simulink model "oppg2b"  (R2024a)
settings: Solver=VariableStepAuto  StartTime=0.0  StopTime=10.0  RelTol=1e-3
settings Model: Creator=Lars André  LastModifiedBy=Lars André

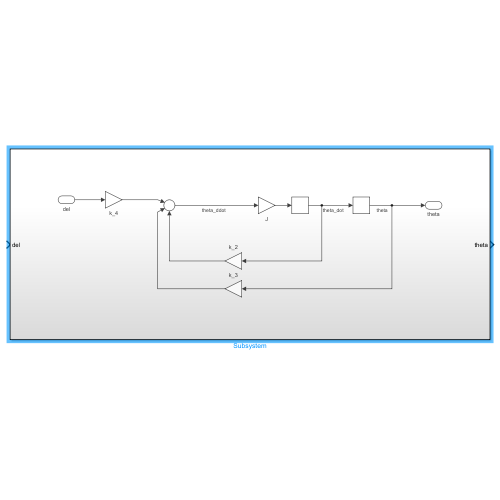
[thumbnail: Simulink's stored preview of the top-level diagram]
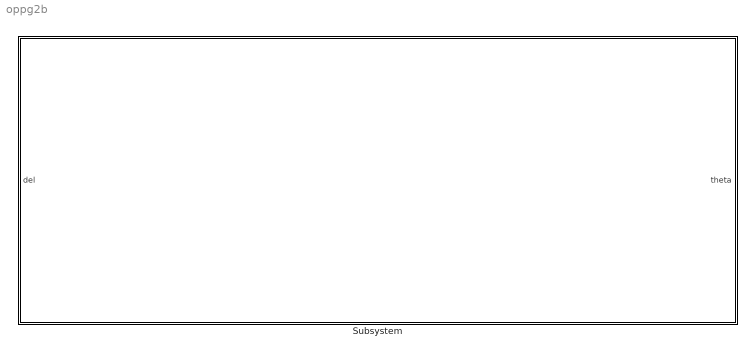
== system oppg2b ==
  Subsystem : Subsystem

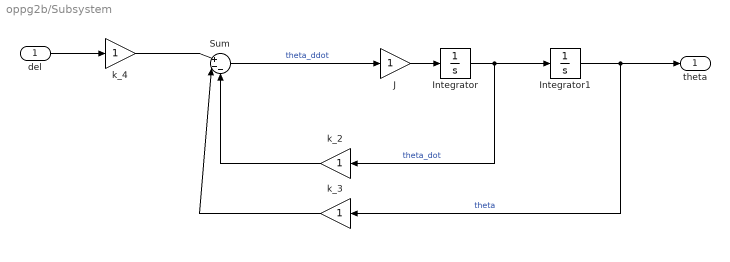
== system oppg2b/Subsystem ==
  del : Inport
  Integrator : Integrator
  Integrator1 : Integrator
  J : Gain
  Sum : Sum  Inputs=|+--
  k_2 : Gain
  k_3 : Gain
  k_4 : Gain
  theta : Outport
  wires:
  Integrator/1 -> Integrator1/1, k_2/1  "theta_dot"
  Integrator1/1 -> theta/1, k_3/1  "theta"
  Sum/1 -> J/1  "theta_ddot"
  del/1 -> k_4/1
  k_4/1 -> Sum/1
  J/1 -> Integrator/1
  k_3/1 -> Sum/2
  k_2/1 -> Sum/3
